simulink model "ControllerSelector"  (R2020a)
settings: Solver=VariableStepAuto  StartTime=0.0  StopTime=10.0  RelTol=1e-3
settings Model: Creator=Sony  LastModifiedBy=Sony

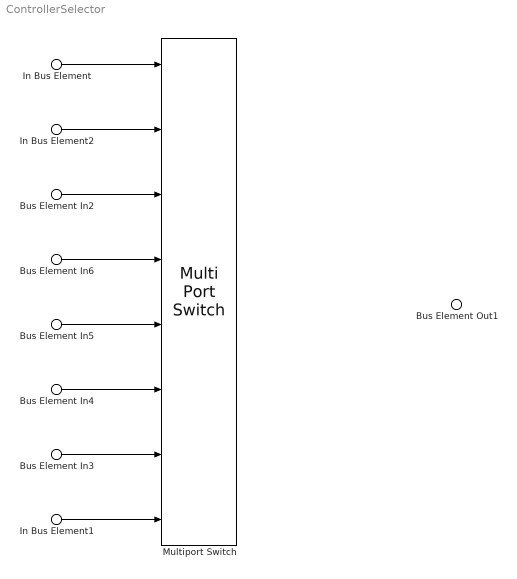
== system ControllerSelector ==
  In Bus Element : Inport  PortName=Selector
  In Bus Element2 : Inport  Port=2  PortName=G1
  Bus Element In2 : Inport  Port=3  PortName=G2
  Bus Element In6 : Inport  Port=4  PortName=G3
  Bus Element In5 : Inport  Port=5  PortName=G4
  Bus Element In4 : Inport  Port=6  PortName=G5
  Bus Element In3 : Inport  Port=7  PortName=G6
  In Bus Element1 : Inport  Port=8  PortName=G7
  Multiport Switch : MultiPortSwitch  Inputs=7
  Bus Element Out1 : Outport  PortName=Gatings
  wires:
  In Bus Element2/1 -> Multiport Switch/2
  Bus Element In2/1 -> Multiport Switch/3
  Bus Element In6/1 -> Multiport Switch/4
  Bus Element In5/1 -> Multiport Switch/5
  Bus Element In4/1 -> Multiport Switch/6
  Bus Element In3/1 -> Multiport Switch/7
  In Bus Element/1 -> Multiport Switch/1
  In Bus Element1/1 -> Multiport Switch/8
